simulink model "HydroEye_6DOF_HITL"  (R2024b)
settings: Solver=VariableStepAuto  StartTime=0.0  StopTime=1200  RelTol=1e-3
undefined symbols (not defined in the file): alpha_vec_Cn0, b, b_ref, beta_vec_Cn0, c, CD, cg, CL, Cl, Clbeta, Clda, Clp, Clr, Cm, Cm0, Cmda, Cmde, Cmq, Cn, Cn0, Cnda, Cnp, Cnr, cp, CX0, CXda, CXde, CY, CYbeta, CYda, CZ0, CZda, CZde, d_ref, Earth, F, Light, mass, MIL, WGS84
libraries: simulink_extras x4, aerolibwind2 x3, aerolibasang x2, aerolibatmos2 x1, aerolibtransform2 x1, shared6dof x1, aerolibadyn x1
settings Model: Creator=01  LastModifiedBy=01
settings OptimizationCC: ReuseModelBlockBuffer=off
settings RTWCC: GPUComputeCapability=3.5

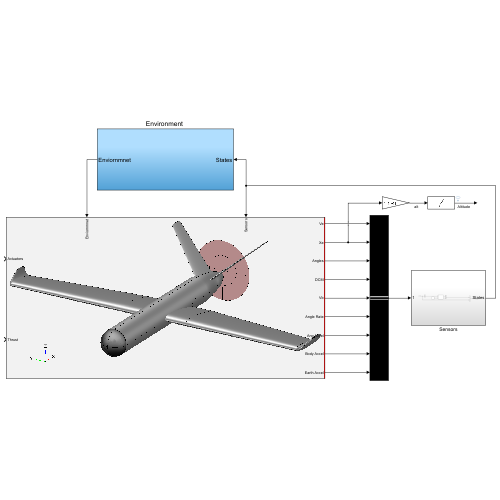
[thumbnail: Simulink's stored preview of the top-level diagram]
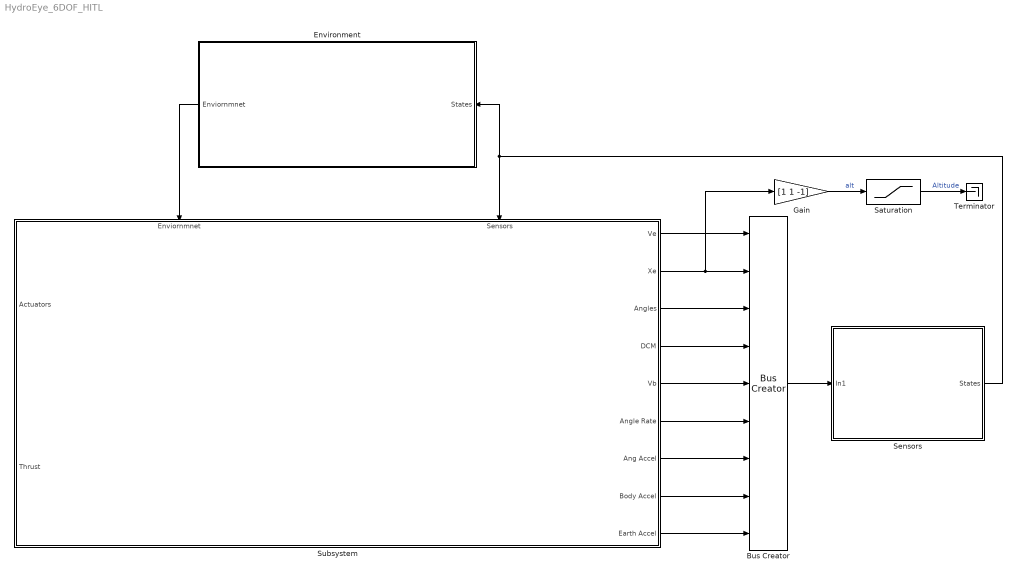
== system HydroEye_6DOF_HITL ==
  Bus Creator : BusCreator  Inputs=9
  "Environment " : Subsystem
      settings: LibrarySourceBlock=|
      | aeroblk_lib_HL20/HL20
      | Airframe/Environment Models
  Gain : Gain  Gain=[1 1 -1]
  Saturation : Saturate  UpperLimit=inf  LowerLimit=0
  Sensors : Subsystem
  Subsystem : Subsystem
      settings: PortSchema="{\"entries\":[{\"content\":{\"sides\":[{\"content\":{\"connectorIds\":[\"In1\",\"In2\"]},\"type\":\"ConnectorPlacement.EquallySpacedRectSide\",\"uuid\":\"55fccbc5-ee7f-44af-8150-33bff5380d0a\"},{\"content\":{\"connectorIds\":[\"Out1\",\"Out2\",\"Out3\",\"Out4\",\"Out5\",\"Out6\",\"Out7\",\"Out8\",\"Out9\"],\"side\":\"RIGHT\"},\"type\":\"ConnectorPlacement.EquallySpacedRectSide\",\"uuid\":\"71396e1b-5d20-4c4e-8e08-515b892d20e7\"},{\"content\":{\"connectorIds\":[\"In3\",\"In4\"],\"side\":\"TOP\"},\"type\":\"ConnectorPlacement.EquallySpacedRectSide\",\"uuid\":\"0174f631-e350-4c9f-98c1-67a3807d9144\"}]},\"type\":\"ConnectorPlacement.EquallySpacedConnector\",\"uuid\":\"de3a6adf-aa37-4a7c-9368-465ba59bc2f3\"}],\"packageUris\":[\"http://schema.mathworks.com/mf0/Connector/R2020b\"],\"version\":\"1.0\"}"
      mask Display: image('s.PNG');
  Terminator : Terminator
  wires:
  Sensors/1(States) -> "Environment "/1(States), Subsystem/4(Sensors)
  Bus Creator/1 -> Sensors/1(In1)
  Gain/1 -> Saturation/1  "alt"
  Saturation/1 -> Terminator/1  "Altitude"
  Subsystem/2(Xe) -> Bus Creator/2, Gain/1
  "Environment "/1(Enviornmnet) -> Subsystem/3(Enviornmnet)
  Subsystem/1(Ve) -> Bus Creator/1
  Subsystem/3(Angles) -> Bus Creator/3
  Subsystem/4(DCM) -> Bus Creator/4
  Subsystem/5(Vb) -> Bus Creator/5
  Subsystem/6(Angle Rate) -> Bus Creator/6
  Subsystem/7(Ang Accel) -> Bus Creator/7
  Subsystem/8(Body Accel) -> Bus Creator/8
  Subsystem/9(Earth Accel) -> Bus Creator/9

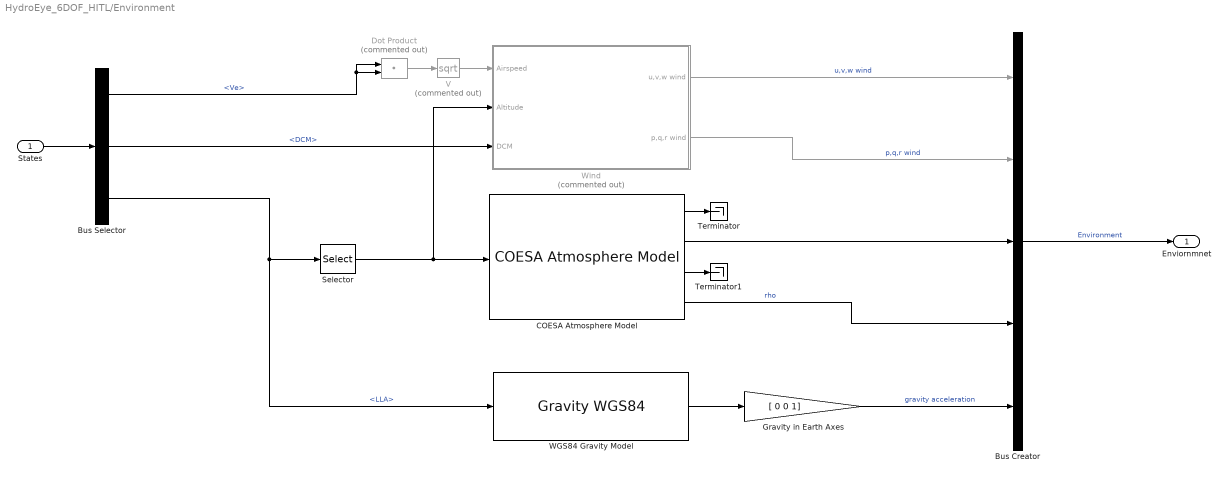
== system HydroEye_6DOF_HITL/Environment  ==
  States : Inport
  Bus Creator : BusCreator  Inputs=5
  Bus Selector : BusSelector  OutputSignals=Raw States.Ve,Raw States.DCM,LLA
  COESA Atmosphere Model : aerolibatmos2/COESA Atmosphere Model  units=Metric (MKS)  spec=1976 COESA-extended U.S. Standard Atmosphere  model=Profile  profile_var=High temperature  profile_percent=10%  profile_alt=5 km (16404 ft)  envelope_var=High temperature  envelope_percent=1%  action=None
      settings: LibrarySourceBlock=|
      | aeroblk_lib_HL20/HL20
      | Airframe/Environment Models/COESA Atmosphere Model
  Dot Product : DotProduct  Commented=on  SaturateOnIntegerOverflow=on  InputSameDT=off  OutDataTypeStr=Inherit: Inherit via internal rule
  Gravity in Earth Axes : Gain  Gain=[ 0 0 1]  SaturateOnIntegerOverflow=on  OutDataTypeStr=Inherit: Same as input  ParamDataTypeStr=Inherit: Same as input
  Selector : Selector  InputPortWidth=3  IndexOptions=Index vector (dialog)  Indices=3  OutputSizes=1
  Terminator : Terminator
  Terminator1 : Terminator
  V : Math  Commented=on  Operator=sqrt  SignedPower=on
  "WGS84 Gravity Model  " : GravityWGS84  action=None
  Wind : Subsystem  Commented=on
  Enviornmnet : Outport
  wires:
  V/1 -> Wind/1(Airspeed)
  "WGS84 Gravity Model  "/1 -> Gravity in Earth Axes/1
  COESA Atmosphere Model/1 -> Terminator/1
  COESA Atmosphere Model/3 -> Terminator1/1
  COESA Atmosphere Model/2 -> Bus Creator/3
  COESA Atmosphere Model/4 -> Bus Creator/4  "rho"
  Selector/1 -> Wind/2(Altitude), COESA Atmosphere Model/1
  Dot Product/1 -> V/1
  Wind/2(p,q,r wind) -> Bus Creator/2  "p,q,r wind"
  Wind/1(u,v,w wind) -> Bus Creator/1  "u,v,w wind"
  Gravity in Earth Axes/1 -> Bus Creator/5  "gravity acceleration"
  States/1 -> Bus Selector/1
  Bus Selector/2 -> Wind/3(DCM)  "<DCM>"
  Bus Selector/1 -> Dot Product/1, Dot Product/2  "<Ve>"
  Bus Selector/3 -> "WGS84 Gravity Model  "/1, Selector/1  "<LLA>"
  Bus Creator/1 -> Enviornmnet/1  "Environment"

== system HydroEye_6DOF_HITL/Sensors ==
  In1 : Inport
  Bus Creator : BusCreator  Inputs=2
  Bus Selector : BusSelector  OutputSignals=Xe
  Constant : Constant  Value=400
  Flat Earth to LLA : aerolibtransform2/Flat Earth to LLA  units=Metric (MKS)  ptype=Earth (WGS84)  F=1/298.257223563  R=6378137  refPosPort=off  LL0=[ 24 46 ]  psi=0
  Mux : Mux  Inputs=2
  States : Outport
  wires:
  In1/1 -> Bus Creator/2, Bus Selector/1  "Raw States"
  Bus Selector/1 -> Flat Earth to LLA/1  "<Xe>"
  Flat Earth to LLA/2 -> Mux/2
  Flat Earth to LLA/1 -> Mux/1
  Mux/1 -> Bus Creator/1  "LLA"
  Bus Creator/1 -> States/1
  Constant/1 -> Flat Earth to LLA/2

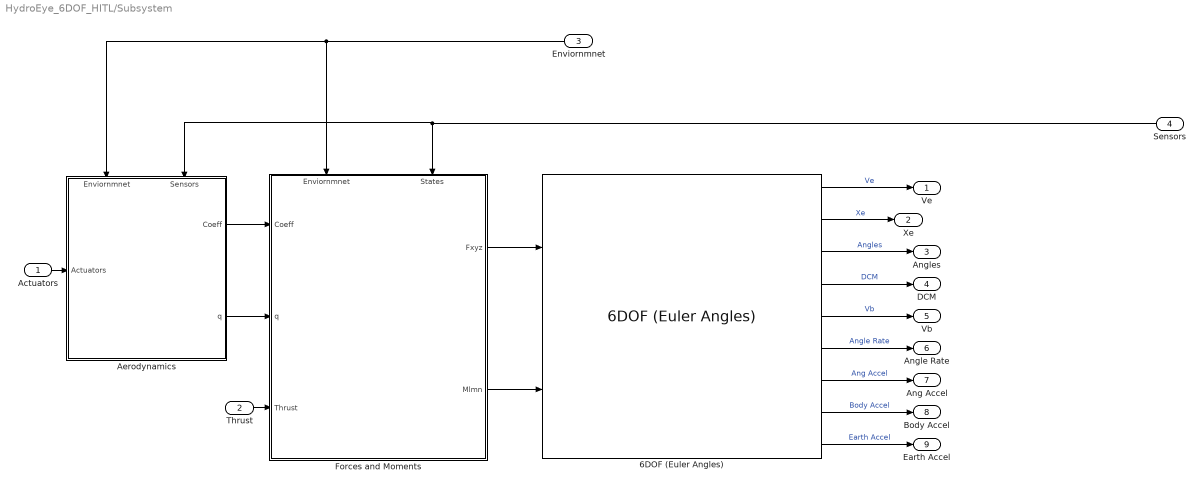
== system HydroEye_6DOF_HITL/Subsystem ==
  Actuators : Inport
  Thrust : Inport  Port=2
  Enviornmnet : Inport  Port=3
  Sensors : Inport  Port=4
  6DOF (Euler Angles) : shared6dof/6DOF (Euler Angles)  units=Metric (MKS)  mtype=Fixed  rep=Euler Angles  xme_0=init.pos  Vm_0=init.V  eul_0=[ 0 deg2rad(2.4) 0 ]  pm_0=[ 0 0 0 ]  mass_0=mass  mass_e=0.5  mass_f=2.0  inertia=I  inertia_e=eye(3)  inertia_f=2*eye(3)  k_quat=1.0  vre_flag=on  abi_flag=on  aMode=aMode  xme_statename=''  Vm_statename=''  eul_statename=''  quat_statename=''  pm_statename=''  mass_statename=''
      settings: LibrarySourceBlock=|
      | aeroblk_lib_HL20/HL20
      | Airframe/6DOF (Euler Angles)
  Aerodynamics : Subsystem
      settings: PortSchema="{\"entries\":[{\"content\":{\"sides\":[{\"content\":{\"connectorIds\":[\"In1\",\"In2\"]},\"type\":\"ConnectorPlacement.EquallySpacedRectSide\",\"uuid\":\"6872a9e6-04cc-43fe-8307-2d3d33caa71d\"},{\"content\":{\"connectorIds\":[],\"side\":\"RIGHT\"},\"type\":\"ConnectorPlacement.EquallySpacedRectSide\",\"uuid\":\"de5f8d1c-5c0e-46cb-94c5-3e4cce4cf93c\"},{\"content\":{\"connectorIds\":[\"In3\"],\"side\":\"TOP\"},\"type\":\"ConnectorPlacement.EquallySpacedRectSide\",\"uuid\":\"d9dd98e0-8ff1-4387-90e5-0ec057a718ca\"},{\"content\":{\"connectorIds\":[\"Out1\",\"Out2\"],\"side\":\"BOTTOM\"},\"type\":\"ConnectorPlacement.EquallySpacedRectSide\",\"uuid\":\"12421dae-0177-4f1a-9b31-64f8981b692b\"}]},\"type\":\"ConnectorPlacement.EquallySpacedConnector\",\"uuid\":\"9e39648a-6fb6-4479-b0ac-1c0f654141e6\"}],\"packageUris\":[\"http://schema.mathworks.com/mf0/Connector/R2020b\"],\"version\":\"1.0\"}"
  Forces and Moments : Subsystem
      settings: PortSchema="{\"entries\":[{\"content\":{\"sides\":[{\"content\":{\"connectorIds\":[\"In1\",\"In2\",\"In3\"]},\"type\":\"ConnectorPlacement.EquallySpacedRectSide\",\"uuid\":\"3fce203a-ae0b-4bce-a87b-30de4173aaf5\"},{\"content\":{\"connectorIds\":[\"Out1\",\"Out2\"],\"side\":\"RIGHT\"},\"type\":\"ConnectorPlacement.EquallySpacedRectSide\",\"uuid\":\"d2fe57eb-25a4-4a3f-81a0-5ad8de127e30\"},{\"content\":{\"connectorIds\":[\"In4\",\"In5\"],\"side\":\"TOP\"},\"type\":\"ConnectorPlacement.EquallySpacedRectSide\",\"uuid\":\"a48e6f39-78f9-49f0-a87f-61fc55168fed\"}]},\"type\":\"ConnectorPlacement.EquallySpacedConnector\",\"uuid\":\"9bf99150-9e27-4a02-9f3a-86824a85a991\"}],\"packageUris\":[\"http://schema.mathworks.com/mf0/Connector/R2020b\"],\"version\":\"1.0\"}"
      settings: LibrarySourceBlock=|
      | aeroblk_lib_HL20/HL20
      | Airframe/Forces and Moments
  Ve : Outport
  Xe : Outport  Port=2
  Angles : Outport  Port=3
  DCM : Outport  Port=4
  Vb : Outport  Port=5
  Angle Rate : Outport  Port=6
  Ang Accel : Outport  Port=7
  Body Accel : Outport  Port=8
  Earth Accel : Outport  Port=9
  wires:
  Aerodynamics/2(q) -> Forces and Moments/2(q)
  Forces and Moments/1(Fxyz) -> 6DOF (Euler Angles)/1
  Sensors/1 -> Aerodynamics/2(Sensors), Forces and Moments/5(States)
  Aerodynamics/1(Coeff) -> Forces and Moments/1(Coeff)
  Enviornmnet/1 -> Forces and Moments/4(Enviornmnet), Aerodynamics/1(Enviornmnet)
  Forces and Moments/2(Mlmn) -> 6DOF (Euler Angles)/2
  Actuators/1 -> Aerodynamics/3(Actuators)
  6DOF (Euler Angles)/4 -> DCM/1  "DCM"
  6DOF (Euler Angles)/2 -> Xe/1  "Xe"
  6DOF (Euler Angles)/1 -> Ve/1  "Ve"
  6DOF (Euler Angles)/3 -> Angles/1  "Angles"
  6DOF (Euler Angles)/6 -> Angle Rate/1  "Angle Rate"
  6DOF (Euler Angles)/8 -> Body Accel/1  "Body Accel"
  6DOF (Euler Angles)/5 -> Vb/1  "Vb"
  6DOF (Euler Angles)/9 -> Earth Accel/1  "Earth Accel"
  6DOF (Euler Angles)/7 -> Ang Accel/1  "Ang Accel"
  Thrust/1 -> Forces and Moments/3(Thrust)

== system HydroEye_6DOF_HITL/Environment /Wind ==
  Airspeed : Inport  Unit=m/s
  Altitude : Inport  Port=2  Unit=m
  DCM : Inport  Port=3
  Discrete Wind Gust Model - On : aerolibwind2/Discrete Wind Gust Model  units=Metric (MKS)  Gx=on  Gy=on  Gz=on  t_0=20  d_m=[120 120 80]  v_m=[3.5 3.0 3.0]
      settings: LibrarySourceBlock=|
      | aeroblk_lib_HL20/HL20
      | Airframe/Environment Models/Wind Models/Discrete Wind Gust Model - On
  Dryden Wind Turbulence Model (Continuous (+q -r)) : aerolibwind2/Dryden Wind Turbulence Model  (Continuous (+q -r))  units=Metric (MKS)  spec=MIL-F-8785C  model=Continuous Dryden (+q -r)  W20=5  Wdeg=0  TurbProb=10^-2 - Light  L_high=533.4  Wingspan=4  ts=0.1  Seed=[23341 23342 23343 23344]  T_on=on
      settings: LibrarySourceBlock=|
      | aeroblk_lib_HL20/HL20
      | Airframe/Environment Models/Wind Models/Dryden Wind Turbulence Model
      | (Continuous (+q -r))
  Sum : Sum  Inputs=+++  InputSameDT=on  SaturateOnIntegerOverflow=on  OutDataTypeStr=Inherit: Same as first input
  Wind Shear Model : aerolibwind2/Wind Shear Model  units=Metric (MKS)  phase=Category C - Terminal Flight Phase  W_20=1  Wdeg=0
      settings: LibrarySourceBlock=|
      | aeroblk_lib_HL20/HL20
      | Airframe/Environment Models/Wind Models/Wind Shear Model
  u,v,w wind : Outport  Unit=m/s  VectorParamsAs1DForOutWhenUnconnected=off
  p,q,r wind : Outport  Port=2  Unit=rad/s  VectorParamsAs1DForOutWhenUnconnected=off
  wires:
  Altitude/1 -> Wind Shear Model/1, Dryden Wind Turbulence Model (Continuous (+q -r))/1
  Dryden Wind Turbulence Model (Continuous (+q -r))/2 -> p,q,r wind/1
  Airspeed/1 -> Discrete Wind Gust Model - On/1, Dryden Wind Turbulence Model (Continuous (+q -r))/2
  DCM/1 -> Wind Shear Model/2, Dryden Wind Turbulence Model (Continuous (+q -r))/3
  Sum/1 -> u,v,w wind/1
  Discrete Wind Gust Model - On/1 -> Sum/3
  Dryden Wind Turbulence Model (Continuous (+q -r))/1 -> Sum/2
  Wind Shear Model/1 -> Sum/1

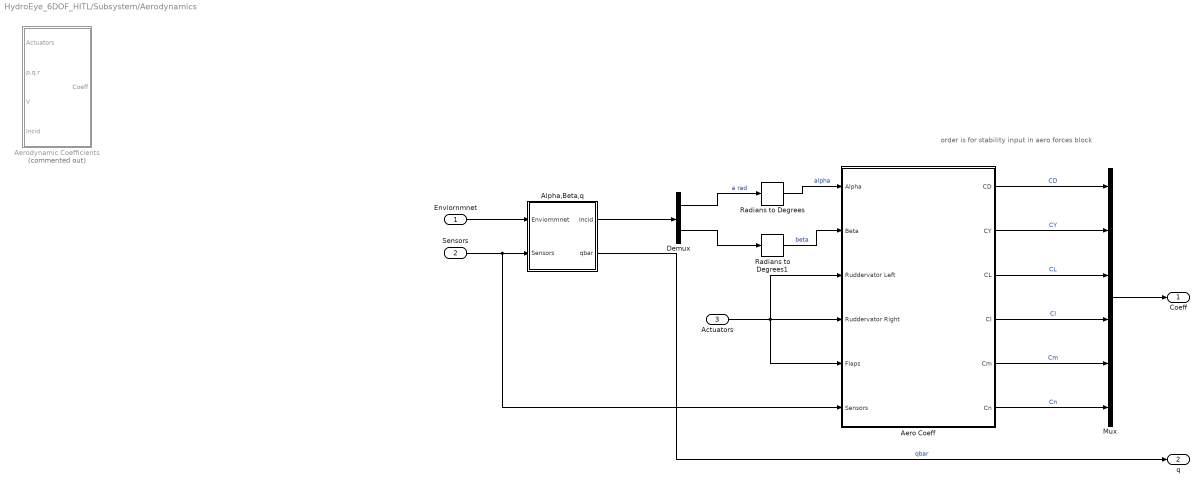
== system HydroEye_6DOF_HITL/Subsystem/Aerodynamics ==
  note: order is for stability input in aero forces block
  Enviornmnet : Inport
  Sensors : Inport  Port=2
  Actuators : Inport  Port=3
  Aero Coeff : Subsystem
  Aerodynamic Coefficients : Subsystem  Commented=on
      settings: LibrarySourceBlock=|
      | aeroblk_lib_HL20/HL20
      | Airframe/Aerodynamic
      | Coefficients
  Alpha,Beta,q : Subsystem
      settings: LibrarySourceBlock=|
      | aeroblk_lib_HL20/HL20
      | Airframe/Alpha,Beta,Mach
  Demux : Demux  Outputs=2
  Mux : Mux  Inputs=6
  Radians to Degrees : simulink_extras/Transformations/Radians to Degrees
  Radians to Degrees1 : simulink_extras/Transformations/Radians to Degrees
  Coeff : Outport
  q : Outport  Port=2
  wires:
  Sensors/1 -> Aero Coeff/6(Sensors), Alpha,Beta,q/2(Sensors)
  Enviornmnet/1 -> Alpha,Beta,q/1(Enviornmnet)
  Alpha,Beta,q/2(qbar) -> q/1  "qbar"
  Mux/1 -> Coeff/1
  Alpha,Beta,q/1(Incid) -> Demux/1
  Aero Coeff/1(CD) -> Mux/1  "CD"
  Aero Coeff/2(CY) -> Mux/2  "CY"
  Aero Coeff/3(CL) -> Mux/3  "CL"
  Aero Coeff/4(Cl) -> Mux/4  "Cl"
  Aero Coeff/5(Cm) -> Mux/5  "Cm"
  Aero Coeff/6(Cn) -> Mux/6  "Cn"
  Radians to Degrees/1 -> Aero Coeff/1(Alpha)  "alpha"
  Radians to Degrees1/1 -> Aero Coeff/2(Beta)  "beta"
  Demux/2 -> Radians to Degrees1/1
  Demux/1 -> Radians to Degrees/1  "a rad"
  Actuators/1 -> Aero Coeff/3(Ruddervator Left), Aero Coeff/4(Ruddervator Right), Aero Coeff/5(Flaps)

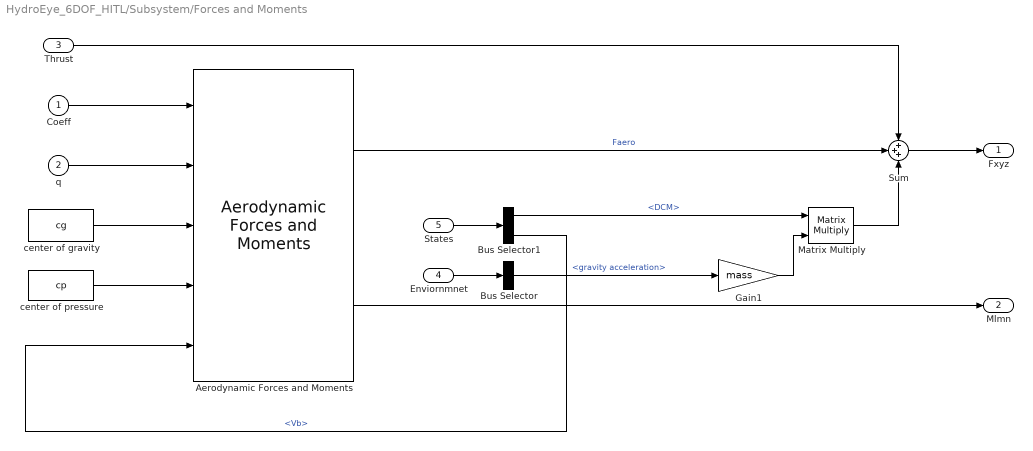
== system HydroEye_6DOF_HITL/Subsystem/Forces and Moments ==
  Coeff : Inport
  q : Inport  Port=2  Unit=Pa
  Thrust : Inport  Port=3
  Enviornmnet : Inport  Port=4
  States : Inport  Port=5
  Aerodynamic Forces and Moments : aerolibadyn/Aerodynamic Forces and Moments   inputAxes=Stability  outputForceAxes=Body  outputMomentAxes=Body  S=Sref  b=b  cbar=c
      settings: LibrarySourceBlock=|
      | aeroblk_lib_HL20/HL20
      | Airframe/Forces and Moments/Aerodynamic
      | Forces and Moments
  Bus Selector : BusSelector  OutputSignals=gravity acceleration
  Bus Selector1 : BusSelector  OutputSignals=Raw States.DCM,Raw States.Vb
  Gain1 : Gain  Gain=mass
  Matrix Multiply : Product  Multiplication=Matrix(*)
  Sum : Sum  Inputs=+++  InputSameDT=on  SaturateOnIntegerOverflow=on  OutDataTypeStr=Inherit: Same as first input
  center of gravity : Constant  Value=cg
  center of pressure : Constant  Value=cp
  Fxyz : Outport
  Mlmn : Outport  Port=2
  wires:
  Coeff/1 -> Aerodynamic Forces and Moments/1
  q/1 -> Aerodynamic Forces and Moments/2
  Sum/1 -> Fxyz/1
  center of gravity/1 -> Aerodynamic Forces and Moments/3
  center of pressure/1 -> Aerodynamic Forces and Moments/4
  Enviornmnet/1 -> Bus Selector/1
  States/1 -> Bus Selector1/1
  Matrix Multiply/1 -> Sum/3
  Bus Selector/1 -> Gain1/1  "<gravity acceleration>"
  Gain1/1 -> Matrix Multiply/2
  Bus Selector1/1 -> Matrix Multiply/1  "<DCM>"
  Thrust/1 -> Sum/1
  Aerodynamic Forces and Moments/1 -> Sum/2  "Faero"
  Aerodynamic Forces and Moments/2 -> Mlmn/1
  Bus Selector1/2 -> Aerodynamic Forces and Moments/5  "<Vb>"

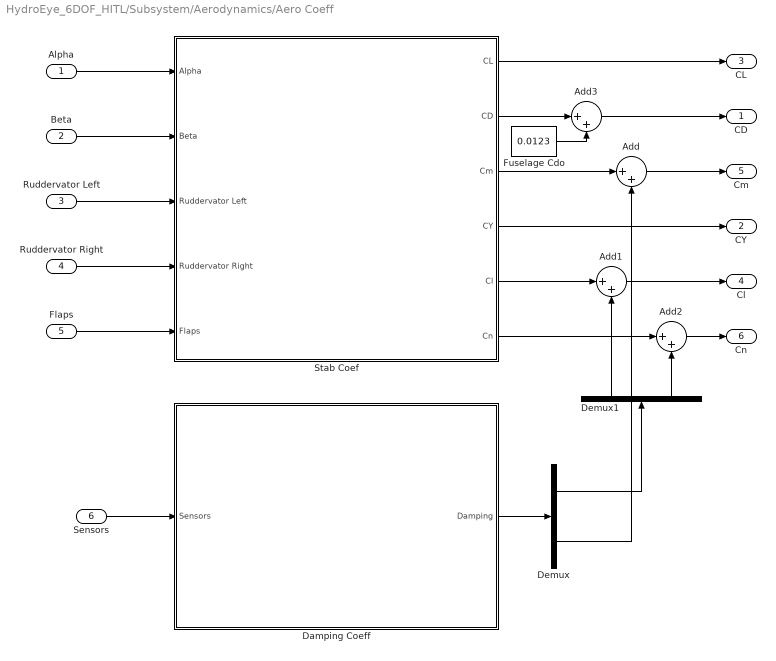
== system HydroEye_6DOF_HITL/Subsystem/Aerodynamics/Aero Coeff ==
  Alpha : Inport
  Beta : Inport  Port=2
  Ruddervator Left : Inport  Port=3
  Ruddervator Right : Inport  Port=4
  Flaps : Inport  Port=5
  Sensors : Inport  Port=6
  Add{,1..3} (4 alike) : Sum  Inputs=|++
  Damping Coeff : Subsystem
  Demux : Demux  Outputs=2
  Demux1 : Demux  Outputs=2
  Fuselage Cdo : Constant  Value=0.0123
  Stab Coef : Subsystem
  CD : Outport
  CY : Outport  Port=2
  CL : Outport  Port=3
  Cl : Outport  Port=4
  Cm : Outport  Port=5
  Cn : Outport  Port=6
  wires:
  Alpha/1 -> Stab Coef/1(Alpha)
  Ruddervator Left/1 -> Stab Coef/3(Ruddervator Left)
  Beta/1 -> Stab Coef/2(Beta)
  Ruddervator Right/1 -> Stab Coef/4(Ruddervator Right)
  Stab Coef/1(CL) -> CL/1
  Stab Coef/4(CY) -> CY/1
  Sensors/1 -> Damping Coeff/1(Sensors)
  Damping Coeff/1(Damping) -> Demux/1
  Stab Coef/3(Cm) -> Add/1
  Add/1 -> Cm/1
  Demux/2 -> Add/2
  Stab Coef/5(Cl) -> Add1/1
  Add1/1 -> Cl/1
  Add2/1 -> Cn/1
  Stab Coef/6(Cn) -> Add2/1
  Demux/1 -> Demux1/1
  Demux1/2 -> Add2/2
  Demux1/1 -> Add1/2
  Stab Coef/2(CD) -> Add3/1
  Add3/1 -> CD/1
  Fuselage Cdo/1 -> Add3/2
  Flaps/1 -> Stab Coef/5(Flaps)

== system HydroEye_6DOF_HITL/Subsystem/Aerodynamics/Aerodynamic Coefficients ==
  Actuators : Inport  Unit=deg
  p,q,r : Inport  Port=2  Unit=rad/second
  V : Inport  Port=3  Unit=m/s
  Incid : Inport  Port=4  Unit=rad
  Actuator Increments : Subsystem
  Body Rate Damping : Subsystem
  Datum Coefficients : Subsystem
  Demux : Demux  Outputs=2
      settings: DisplayOption=none
  Sum1 : Sum  Inputs=+++  InputSameDT=on  SaturateOnIntegerOverflow=on  OutDataTypeStr=Inherit: Same as first input
  Coeff : Outport  InitialOutput=0  VectorParamsAs1DForOutWhenUnconnected=off
  wires:
  Demux/1 -> Datum Coefficients/1(Alpha), Actuator Increments/1(Alpha), Body Rate Damping/3(Alpha)
  p,q,r/1 -> Body Rate Damping/2(p,q,r)
  Incid/1 -> Demux/1
  Actuators/1 -> Actuator Increments/2("Actuator Deflections ")
  Sum1/1 -> Coeff/1
  Datum Coefficients/1(cl) -> Sum1/2
  Demux/2 -> Datum Coefficients/2(Beta)
  V/1 -> Body Rate Damping/1(V)
  Body Rate Damping/1(cl) -> Sum1/1
  Actuator Increments/1(cl) -> Sum1/3

== system HydroEye_6DOF_HITL/Subsystem/Aerodynamics/Alpha,Beta,q ==
  Enviornmnet : Inport
  Sensors : Inport  Port=2
  Bus Selector : BusSelector  OutputSignals=rho
  Bus Selector1 : BusSelector  OutputSignals=Raw States.Vb
  Dynamic Pressure : aerolibasang/Dynamic Pressure
      settings: LibrarySourceBlock=|
      | aeroblk_lib_HL20/HL20
      | Airframe/Alpha,Beta,Mach/Dynamic Pressure
  "Incidence, Sideslip & Airspeed" : aerolibasang/Incidence, Sideslip, & Airspeed
      settings: LibrarySourceBlock=|
      | aeroblk_lib_HL20/HL20
      | Airframe/Alpha,Beta,Mach/Incidence, Sideslip
      | & Airspeed
  Mux : Mux  Inputs=2
  Incid : Outport  Unit=rad  VectorParamsAs1DForOutWhenUnconnected=off
  qbar : Outport  Port=2  Unit=Pa  InitialOutput=0  VectorParamsAs1DForOutWhenUnconnected=off
  wires:
  "Incidence, Sideslip & Airspeed"/1 -> Mux/1  "Alpha"
  Mux/1 -> Incid/1
  "Incidence, Sideslip & Airspeed"/2 -> Mux/2  "Beta"
  Dynamic Pressure/1 -> qbar/1
  Enviornmnet/1 -> Bus Selector/1
  Bus Selector/1 -> Dynamic Pressure/2  "<rho>"
  Sensors/1 -> Bus Selector1/1
  Bus Selector1/1 -> "Incidence, Sideslip & Airspeed"/1, Dynamic Pressure/1  "<Vb>"

== system HydroEye_6DOF_HITL/Subsystem/Aerodynamics/Aero Coeff/Damping Coeff ==
  Sensors : Inport
  Bus Selector : BusSelector  OutputSignals=Raw States.Angle Rate,Raw States.Vb
  Mux : Mux  Inputs=2
  p & r : Subsystem
  q : Subsystem
  Damping : Outport
  wires:
  Sensors/1 -> Bus Selector/1
  q/1(pitch rate damping) -> Mux/2
  Mux/1 -> Damping/1
  p & r/1(roll rate damping) -> Mux/1
  Bus Selector/1 -> q/1(<Angle Rate>), p & r/1(<Angle Rate>)  "<Angle Rate>"
  Bus Selector/2 -> q/2(<Vb>), p & r/2(<Vb>)  "<Vb>"

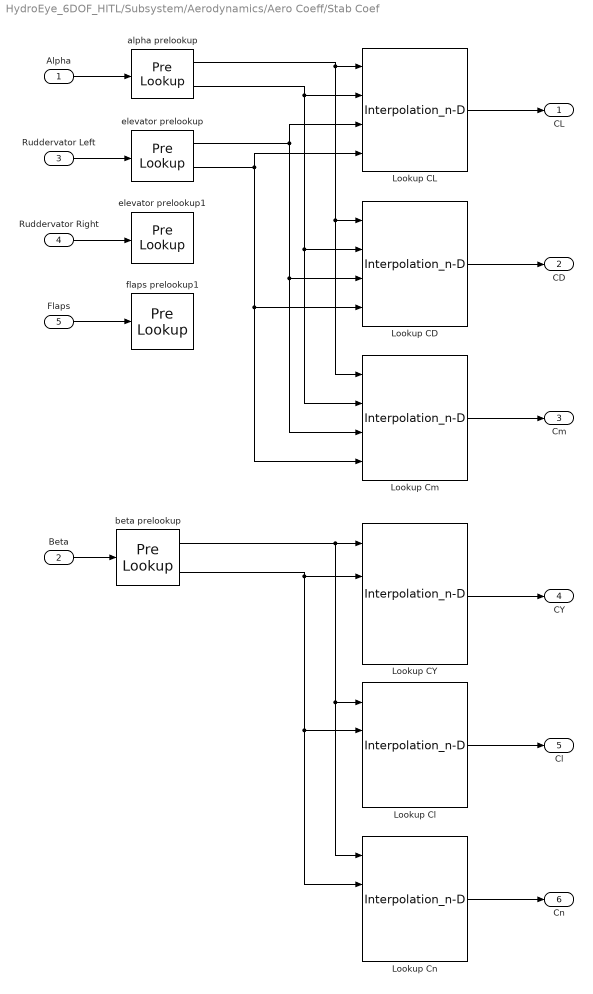
== system HydroEye_6DOF_HITL/Subsystem/Aerodynamics/Aero Coeff/Stab Coef ==
  Alpha : Inport
  Beta : Inport  Port=2
  Ruddervator Left : Inport  Port=3
  Ruddervator Right : Inport  Port=4
  Flaps : Inport  Port=5
  Lookup CD : Interpolation_n-D  Table=CD  InternalRulePriority=Speed
  Lookup CL : Interpolation_n-D  Table=CL  InternalRulePriority=Speed
  Lookup CY : Interpolation_n-D  Table=CY  InternalRulePriority=Speed
  Lookup Cl : Interpolation_n-D  Table=Cl  InternalRulePriority=Speed
  Lookup Cm : Interpolation_n-D  Table=Cm  InternalRulePriority=Speed
  Lookup Cn : Interpolation_n-D  Table=Cn  InternalRulePriority=Speed
  alpha prelookup : PreLookup  BreakpointsData=alpha  BeginIndexSearchUsingPreviousIndexResult=on  ExtrapMethod=Linear
  beta prelookup : PreLookup  BreakpointsData=beta  ExtrapMethod=Linear
  elevator prelookup : PreLookup  BreakpointsData=elevator  ExtrapMethod=Linear
  elevator prelookup1 : PreLookup  BreakpointsData=elevator  ExtrapMethod=Linear
  flaps prelookup1 : PreLookup  BreakpointsData=elevator  ExtrapMethod=Linear
  CL : Outport
  CD : Outport  Port=2
  Cm : Outport  Port=3
  CY : Outport  Port=4
  Cl : Outport  Port=5
  Cn : Outport  Port=6
  wires:
  beta prelookup/2 -> Lookup Cn/2, Lookup Cl/2, Lookup CY/2
  alpha prelookup/1 -> Lookup Cm/1, Lookup CD/1, Lookup CL/1
  beta prelookup/1 -> Lookup Cn/1, Lookup Cl/1, Lookup CY/1
  elevator prelookup/1 -> Lookup CL/3, Lookup Cm/3, Lookup CD/3
  Lookup Cn/1 -> Cn/1
  Alpha/1 -> alpha prelookup/1
  alpha prelookup/2 -> Lookup Cm/2, Lookup CD/2, Lookup CL/2
  elevator prelookup/2 -> Lookup Cm/4, Lookup CD/4, Lookup CL/4
  Lookup CL/1 -> CL/1
  Beta/1 -> beta prelookup/1
  Lookup Cm/1 -> Cm/1
  Ruddervator Left/1 -> elevator prelookup/1
  Lookup CY/1 -> CY/1
  Lookup Cl/1 -> Cl/1
  Lookup CD/1 -> CD/1
  Flaps/1 -> flaps prelookup1/1
  Ruddervator Right/1 -> elevator prelookup1/1

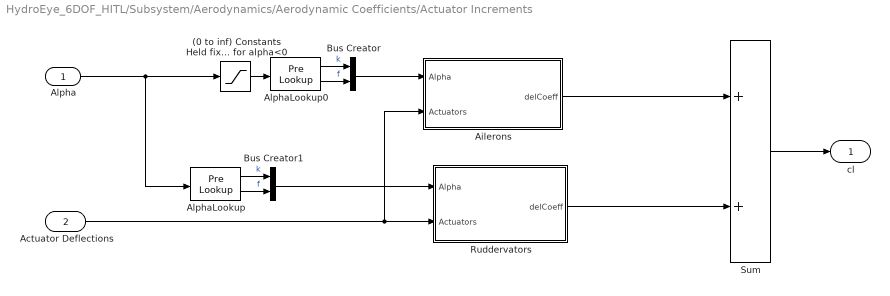
== system HydroEye_6DOF_HITL/Subsystem/Aerodynamics/Aerodynamic Coefficients/Actuator Increments ==
  Alpha : Inport  Unit=deg
  "Actuator Deflections " : Inport  Port=2  Unit=deg
  (0 to inf) Constants Held fixed for alpha<0 : Saturate  UpperLimit=inf  LowerLimit=0
  Ailerons : Subsystem
  AlphaLookup : PreLookup  BreakpointsData=alpha_vec_0  BeginIndexSearchUsingPreviousIndexResult=on  ExtrapMethod=Linear
  AlphaLookup0 : PreLookup  BreakpointsData=alpha_vec_0  BeginIndexSearchUsingPreviousIndexResult=on  ExtrapMethod=Linear
  Bus Creator : BusCreator  Inputs=2
  Bus Creator1 : BusCreator  Inputs=2
  Ruddervators : Subsystem
  Sum : Sum  InputSameDT=on  SaturateOnIntegerOverflow=on  OutDataTypeStr=Inherit: Same as first input
  cl : Outport  InitialOutput=0  VectorParamsAs1DForOutWhenUnconnected=off
  wires:
  Bus Creator/1 -> Ailerons/1(Alpha)
  (0 to inf) Constants Held fixed for alpha<0/1 -> AlphaLookup0/1
  "Actuator Deflections "/1 -> Ailerons/2(Actuators), Ruddervators/2(Actuators)
  Alpha/1 -> (0 to inf) Constants Held fixed for alpha<0/1, AlphaLookup/1
  Ailerons/1(delCoeff) -> Sum/1
  Ruddervators/1(delCoeff) -> Sum/2
  Sum/1 -> cl/1
  Bus Creator1/1 -> Ruddervators/1(Alpha)
  AlphaLookup0/1 -> Bus Creator/1  "k"
  AlphaLookup0/2 -> Bus Creator/2  "f"
  AlphaLookup/1 -> Bus Creator1/1  "k"
  AlphaLookup/2 -> Bus Creator1/2  "f"

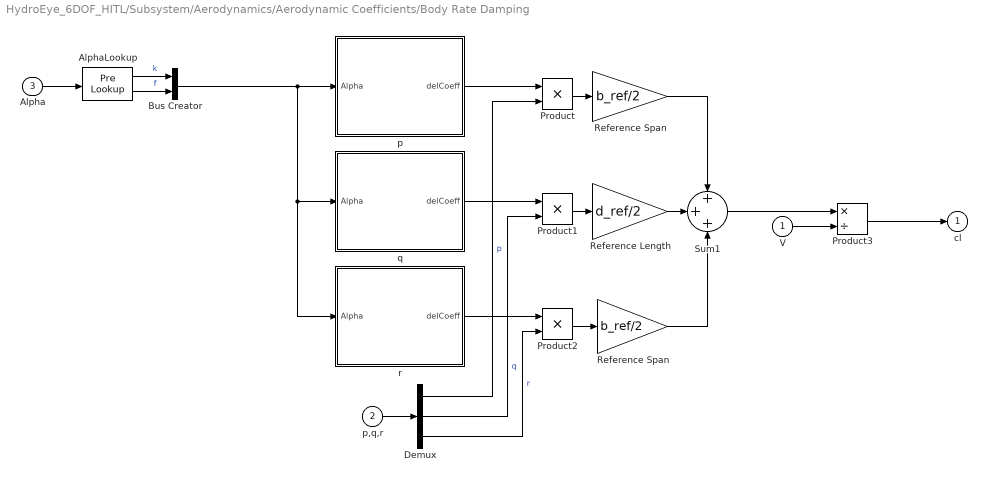
== system HydroEye_6DOF_HITL/Subsystem/Aerodynamics/Aerodynamic Coefficients/Body Rate Damping ==
  V : Inport  Unit=m/s
  p,q,r : Inport  Port=2  Unit=rad/second
  Alpha : Inport  Port=3  Unit=deg
  AlphaLookup : PreLookup  BreakpointsData=alpha_vec_damping  BeginIndexSearchUsingPreviousIndexResult=on  ExtrapMethod=Linear
  Bus Creator : BusCreator  Inputs=2
  Demux : Demux  Outputs=3
      settings: DisplayOption=none
  Product : Product  InputSameDT=on  SaturateOnIntegerOverflow=on  OutDataTypeStr=Inherit: Same as first input
  Product1 : Product  InputSameDT=on  SaturateOnIntegerOverflow=on  OutDataTypeStr=Inherit: Same as first input
  Product2 : Product  InputSameDT=on  SaturateOnIntegerOverflow=on  OutDataTypeStr=Inherit: Same as first input
  Product3 : Product  Inputs=*/  InputSameDT=on  SaturateOnIntegerOverflow=on  OutDataTypeStr=Inherit: Same as first input
  Reference Length : Gain  Gain=d_ref/2  SaturateOnIntegerOverflow=on  OutDataTypeStr=Inherit: Same as input  ParamDataTypeStr=Inherit: Same as input
  Reference Span : Gain  Gain=b_ref/2  SaturateOnIntegerOverflow=on  OutDataTypeStr=Inherit: Same as input  ParamDataTypeStr=Inherit: Same as input
  "Reference Span " : Gain  Gain=b_ref/2  SaturateOnIntegerOverflow=on  OutDataTypeStr=Inherit: Same as input  ParamDataTypeStr=Inherit: Same as input
  Sum1 : Sum  Inputs=+++  InputSameDT=on  SaturateOnIntegerOverflow=on  OutDataTypeStr=Inherit: Same as first input
  p : Subsystem
  q : Subsystem
  r : Subsystem
  cl : Outport  InitialOutput=0  VectorParamsAs1DForOutWhenUnconnected=off
  wires:
  Alpha/1 -> AlphaLookup/1
  p/1(delCoeff) -> Product/1
  q/1(delCoeff) -> Product1/1
  p,q,r/1 -> Demux/1
  Demux/1 -> Product/2  "p"
  Demux/2 -> Product1/2  "q"
  Demux/3 -> Product2/2  "r"
  Sum1/1 -> Product3/1
  V/1 -> Product3/2
  Product3/1 -> cl/1
  Product1/1 -> Reference Length/1
  Product2/1 -> "Reference Span "/1
  Product/1 -> Reference Span/1
  r/1(delCoeff) -> Product2/1
  Bus Creator/1 -> r/1(Alpha), q/1(Alpha), p/1(Alpha)
  Reference Length/1 -> Sum1/2
  Reference Span/1 -> Sum1/1
  "Reference Span "/1 -> Sum1/3
  AlphaLookup/1 -> Bus Creator/1  "k"
  AlphaLookup/2 -> Bus Creator/2  "f"

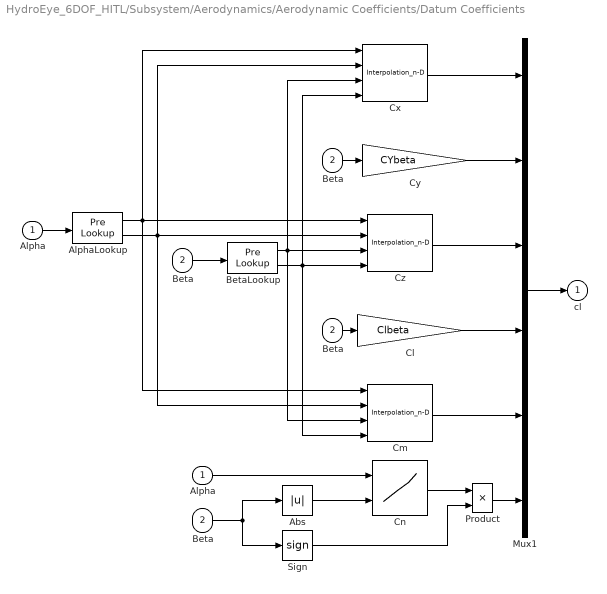
== system HydroEye_6DOF_HITL/Subsystem/Aerodynamics/Aerodynamic Coefficients/Datum Coefficients ==
  Alpha : Inport  Unit=deg
  Beta : Inport  Port=2  Unit=deg
  " Cn" : Lookup_n-D  BreakpointsForDimension1=alpha_vec_Cn0  BreakpointsForDimension2=beta_vec_Cn0  Table=Cn0  InternalRulePriority=Speed  RndMeth=Simplest
      settings: InputPortMap=u0,u1
  " Beta" : InportShadow  Port=2  Unit=deg
  " Beta " : InportShadow  Port=2  Unit=deg
  Abs : Abs
  "Alpha " : InportShadow  Unit=deg
  AlphaLookup : PreLookup  BreakpointsData=alpha_vec_0  BeginIndexSearchUsingPreviousIndexResult=on  ExtrapMethod=Linear
  "Beta " : InportShadow  Port=2  Unit=deg
  BetaLookup : PreLookup  BreakpointsData=beta_vec_0  BeginIndexSearchUsingPreviousIndexResult=on  ExtrapMethod=Linear
  Cl : Gain  Gain=Clbeta  SaturateOnIntegerOverflow=on  OutDataTypeStr=Inherit: Same as input  ParamDataTypeStr=Inherit: Same as input
  Cm : Interpolation_n-D  Table=Cm0'  RemoveProtectionIndex=on
  Cx : Interpolation_n-D  Table=CX0'  RemoveProtectionIndex=on
  Cy : Gain  Gain=CYbeta  SaturateOnIntegerOverflow=on  OutDataTypeStr=Inherit: Same as input  ParamDataTypeStr=Inherit: Same as input
  Cz : Interpolation_n-D  Table=CZ0'  RemoveProtectionIndex=on
  Mux1 : Mux  Inputs=6
  Product : Product  InputSameDT=on  SaturateOnIntegerOverflow=on  OutDataTypeStr=Inherit: Same as first input
  Sign : Signum
  cl : Outport  InitialOutput=0  VectorParamsAs1DForOutWhenUnconnected=off
  wires:
  Sign/1 -> Product/2
  " Cn"/1 -> Product/1
  Product/1 -> Mux1/6
  Abs/1 -> " Cn"/2
  Mux1/1 -> cl/1
  Cx/1 -> Mux1/1
  Cz/1 -> Mux1/3
  Cm/1 -> Mux1/5
  Cy/1 -> Mux1/2
  Cl/1 -> Mux1/4
  Alpha/1 -> AlphaLookup/1
  Beta/1 -> BetaLookup/1
  AlphaLookup/1 -> Cz/1, Cm/1, Cx/1
  BetaLookup/1 -> Cz/3, Cx/3, Cm/3
  AlphaLookup/2 -> Cx/2, Cm/2, Cz/2
  "Beta "/1 -> Cy/1
  "Alpha "/1 -> " Cn"/1
  " Beta"/1 -> Abs/1, Sign/1
  " Beta "/1 -> Cl/1
  BetaLookup/2 -> Cz/4, Cx/4, Cm/4

== system HydroEye_6DOF_HITL/Subsystem/Aerodynamics/Aero Coeff/Damping Coeff/p & r ==
  <Angle Rate> : Inport
  <Vb> : Inport  Port=2
  Constant : Constant  Value=[Clp 0 Clr; Cnp 0 Cnr]
  Divide : Product  Inputs=*/
  Dot Product : DotProduct  OutDataTypeStr=Inherit: Inherit via internal rule
  Gain1 : Gain  Gain=b
  Gain2 : Gain  Gain=2
  Matrix Multiply : Product  Multiplication=Matrix(*)
  Radians to Degrees : simulink_extras/Transformations/Radians to Degrees
  Sqrt : Sqrt
  roll rate damping : Outport
  wires:
  Gain2/1 -> Divide/2
  Matrix Multiply/1 -> Gain1/1
  Gain1/1 -> Divide/1
  Divide/1 -> roll rate damping/1  "roll rate damping"
  Constant/1 -> Matrix Multiply/1
  <Vb>/1 -> Dot Product/1, Dot Product/2
  Dot Product/1 -> Sqrt/1
  Sqrt/1 -> Gain2/1
  <Angle Rate>/1 -> Radians to Degrees/1
  Radians to Degrees/1 -> Matrix Multiply/2

== system HydroEye_6DOF_HITL/Subsystem/Aerodynamics/Aero Coeff/Damping Coeff/q ==
  <Angle Rate> : Inport
  <Vb> : Inport  Port=2
  Divide : Product  Inputs=*/
  Dot Product : DotProduct  OutDataTypeStr=Inherit: Inherit via internal rule
  Gain : Gain  Gain=Cmq
  Gain1 : Gain  Gain=c
  Gain2 : Gain  Gain=2
  Radians to Degrees : simulink_extras/Transformations/Radians to Degrees
  Selector : Selector  InputPortWidth=3  IndexOptions=Index vector (dialog)  Indices=2  OutputSizes=1
  pitch rate damping : Outport
  wires:
  Selector/1 -> Gain/1
  Gain2/1 -> Divide/2
  Gain/1 -> Gain1/1
  Gain1/1 -> Divide/1
  Divide/1 -> pitch rate damping/1  "pitch rate damping"
  <Vb>/1 -> Dot Product/1, Dot Product/2
  Dot Product/1 -> Gain2/1
  <Angle Rate>/1 -> Radians to Degrees/1
  Radians to Degrees/1 -> Selector/1

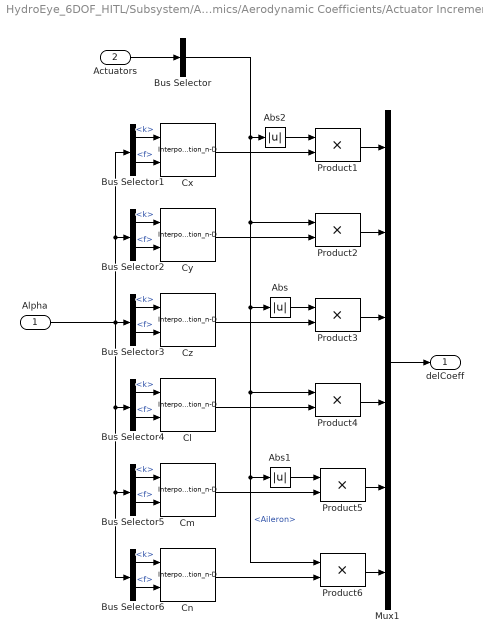
== system HydroEye_6DOF_HITL/Subsystem/Aerodynamics/Aerodynamic Coefficients/Actuator Increments/Ailerons ==
  Alpha : Inport
  Actuators : Inport  Port=2
  Abs : Abs
  Abs1 : Abs
  Abs2 : Abs
  Bus Selector : BusSelector  OutputSignals=Aileron
  Bus Selector{1..6} (6 alike) : BusSelector  OutputSignals=k,f
  Cl : Interpolation_n-D  NumberOfTableDimensions=1  Table=Clda  RemoveProtectionIndex=on
      settings: InputPortMap=u0,u1
  Cm : Interpolation_n-D  NumberOfTableDimensions=1  Table=Cmda  RemoveProtectionIndex=on
      settings: InputPortMap=u0,u1
  Cn : Interpolation_n-D  NumberOfTableDimensions=1  Table=Cnda  RemoveProtectionIndex=on
      settings: InputPortMap=u0,u1
  Cx : Interpolation_n-D  NumberOfTableDimensions=1  Table=CXda  RemoveProtectionIndex=on
      settings: InputPortMap=u0,u1
  Cy : Interpolation_n-D  NumberOfTableDimensions=1  Table=CYda  RemoveProtectionIndex=on
      settings: InputPortMap=u0,u1
  Cz : Interpolation_n-D  NumberOfTableDimensions=1  Table=CZda  RemoveProtectionIndex=on
      settings: InputPortMap=u0,u1
  Mux1 : Mux  Inputs=6
  Product{1..6} (6 alike) : Product  InputSameDT=on  SaturateOnIntegerOverflow=on  OutDataTypeStr=Inherit: Same as first input
  delCoeff : Outport  VectorParamsAs1DForOutWhenUnconnected=off
  wires:
  Actuators/1 -> Bus Selector/1
  Mux1/1 -> delCoeff/1
  Product1/1 -> Mux1/1
  Cx/1 -> Product1/2
  Product2/1 -> Mux1/2
  Cy/1 -> Product2/2
  Product3/1 -> Mux1/3
  Cz/1 -> Product3/2
  Cl/1 -> Product4/2
  Product4/1 -> Mux1/4
  Cm/1 -> Product5/2
  Product5/1 -> Mux1/5
  Cn/1 -> Product6/2
  Product6/1 -> Mux1/6
  Bus Selector/1 -> Product6/1, Abs1/1, Product4/1, Abs/1, Product2/1, Abs2/1  "<Aileron>"
  Abs/1 -> Product3/1
  Abs1/1 -> Product5/1
  Abs2/1 -> Product1/1
  Alpha/1 -> Bus Selector1/1, Bus Selector2/1, Bus Selector5/1, Bus Selector6/1, Bus Selector4/1, Bus Selector3/1
  Bus Selector1/1 -> Cx/1  "<k>"
  Bus Selector1/2 -> Cx/2  "<f>"
  Bus Selector2/1 -> Cy/1  "<k>"
  Bus Selector2/2 -> Cy/2  "<f>"
  Bus Selector3/1 -> Cz/1  "<k>"
  Bus Selector3/2 -> Cz/2  "<f>"
  Bus Selector4/1 -> Cl/1  "<k>"
  Bus Selector4/2 -> Cl/2  "<f>"
  Bus Selector5/1 -> Cm/1  "<k>"
  Bus Selector5/2 -> Cm/2  "<f>"
  Bus Selector6/1 -> Cn/1  "<k>"
  Bus Selector6/2 -> Cn/2  "<f>"

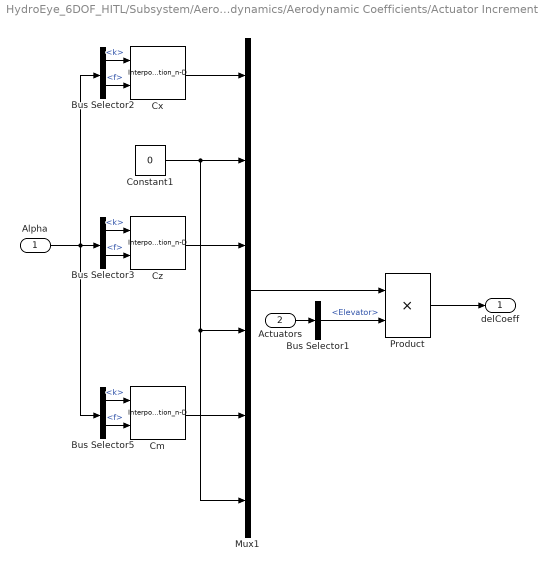
== system HydroEye_6DOF_HITL/Subsystem/Aerodynamics/Aerodynamic Coefficients/Actuator Increments/Ruddervators ==
  Alpha : Inport
  Actuators : Inport  Port=2
  Bus Selector1 : BusSelector  OutputSignals=Elevator
  Bus Selector2 : BusSelector  OutputSignals=k,f
  Bus Selector3 : BusSelector  OutputSignals=k,f
  Bus Selector5 : BusSelector  OutputSignals=k,f
  Cm : Interpolation_n-D  NumberOfTableDimensions=1  Table=Cmde  RemoveProtectionIndex=on
      settings: InputPortMap=u0,u1
  Constant1 : Constant  Value=0
  Cx : Interpolation_n-D  NumberOfTableDimensions=1  Table=CXde  RemoveProtectionIndex=on
      settings: InputPortMap=u0,u1
  Cz : Interpolation_n-D  NumberOfTableDimensions=1  Table=CZde  RemoveProtectionIndex=on
      settings: InputPortMap=u0,u1
  Mux1 : Mux  Inputs=6
  Product : Product  InputSameDT=on  SaturateOnIntegerOverflow=on  OutDataTypeStr=Inherit: Same as first input
  delCoeff : Outport  VectorParamsAs1DForOutWhenUnconnected=off
  wires:
  Product/1 -> delCoeff/1
  Mux1/1 -> Product/1
  Alpha/1 -> Bus Selector2/1, Bus Selector3/1, Bus Selector5/1
  Cx/1 -> Mux1/1
  Cz/1 -> Mux1/3
  Cm/1 -> Mux1/5
  Constant1/1 -> Mux1/2, Mux1/4, Mux1/6
  Actuators/1 -> Bus Selector1/1
  Bus Selector1/1 -> Product/2  "<Elevator>"
  Bus Selector2/1 -> Cx/1  "<k>"
  Bus Selector2/2 -> Cx/2  "<f>"
  Bus Selector3/1 -> Cz/1  "<k>"
  Bus Selector3/2 -> Cz/2  "<f>"
  Bus Selector5/1 -> Cm/1  "<k>"
  Bus Selector5/2 -> Cm/2  "<f>"

== system HydroEye_6DOF_HITL/Subsystem/Aerodynamics/Aerodynamic Coefficients/Body Rate Damping/p ==
  Alpha : Inport
  Bus Selector : BusSelector  OutputSignals=k,f
  Bus Selector1 : BusSelector  OutputSignals=k,f
  Cl : Interpolation_n-D  NumberOfTableDimensions=1  Table=Clp  RemoveProtectionIndex=on
      settings: InputPortMap=u0,u1
  Cn : Interpolation_n-D  NumberOfTableDimensions=1  Table=Cnp  RemoveProtectionIndex=on
      settings: InputPortMap=u0,u1
  Constant1 : Constant  Value=0
  Mux1 : Mux  Inputs=6
  delCoeff : Outport  VectorParamsAs1DForOutWhenUnconnected=off
  wires:
  Mux1/1 -> delCoeff/1
  Constant1/1 -> Mux1/1, Mux1/5, Mux1/3, Mux1/2  "Cxp"
  Cn/1 -> Mux1/6
  Cl/1 -> Mux1/4  "Cl"
  Alpha/1 -> Bus Selector/1, Bus Selector1/1
  Bus Selector/1 -> Cl/1  "<k>"
  Bus Selector/2 -> Cl/2  "<f>"
  Bus Selector1/1 -> Cn/1  "<k>"
  Bus Selector1/2 -> Cn/2  "<f>"

== system HydroEye_6DOF_HITL/Subsystem/Aerodynamics/Aerodynamic Coefficients/Body Rate Damping/q ==
  Alpha : Inport
  Bus Selector1 : BusSelector  OutputSignals=k,f
  Cmq : Interpolation_n-D  NumberOfTableDimensions=1  Table=Cmq  RemoveProtectionIndex=on
      settings: InputPortMap=u0,u1
  Constant3 : Constant  Value=0
  Mux1 : Mux  Inputs=6
  delCoeff : Outport  VectorParamsAs1DForOutWhenUnconnected=off
  wires:
  Cmq/1 -> Mux1/5
  Constant3/1 -> Mux1/1, Mux1/2, Mux1/3, Mux1/6, Mux1/4
  Mux1/1 -> delCoeff/1
  Alpha/1 -> Bus Selector1/1
  Bus Selector1/1 -> Cmq/1  "<k>"
  Bus Selector1/2 -> Cmq/2  "<f>"

== system HydroEye_6DOF_HITL/Subsystem/Aerodynamics/Aerodynamic Coefficients/Body Rate Damping/r ==
  Alpha : Inport
  Bus Selector : BusSelector  OutputSignals=k,f
  Bus Selector1 : BusSelector  OutputSignals=k,f
  Cl : Interpolation_n-D  NumberOfTableDimensions=1  Table=Clr  RemoveProtectionIndex=on
      settings: InputPortMap=u0,u1
  Cn : Interpolation_n-D  NumberOfTableDimensions=1  Table=Cnr  RemoveProtectionIndex=on
      settings: InputPortMap=u0,u1
  Constant : Constant  Value=0
  Mux1 : Mux  Inputs=6
  delCoeff : Outport  VectorParamsAs1DForOutWhenUnconnected=off
  wires:
  Cn/1 -> Mux1/6
  Cl/1 -> Mux1/4  "Cl"
  Constant/1 -> Mux1/1, Mux1/2, Mux1/5, Mux1/3  "Cxr"
  Mux1/1 -> delCoeff/1
  Alpha/1 -> Bus Selector1/1, Bus Selector/1
  Bus Selector/1 -> Cl/1  "<k>"
  Bus Selector/2 -> Cl/2  "<f>"
  Bus Selector1/1 -> Cn/1  "<k>"
  Bus Selector1/2 -> Cn/2  "<f>"
